simulink model "SAID"  (R2020a)
settings: Solver=ode45  StartTime=0  StopTime=15  FixedStep=0.002  RelTol=1e-3  AbsTol=1e-6
libraries: simulink x2, Solver_SF x1
settings Model: ExtModeTrigMode=oneshot  ExtModeArmWhenConnect=off  Creator=ywata  LastModifiedBy=wcbos
settings SolverCC: AutoScaleAbsTol=off  AlgebraicLoopSolver=LineSearch
settings DataIOCC: SaveFormat=Array  ReturnWorkspaceOutputs=off  SignalLoggingName=sigsOut
settings OptimizationCC: BlockReduction=off  BooleanDataType=off  ExpressionDepthLimit=2147483647  LifeSpan=inf
settings DebuggingCC: SaveWithParameterizedLinksMsg=none  UnderspecifiedInitializationDetection=Classic  MergeDetectMultiDrivingBlocksExec=none  SignalResolutionControl=TryResolveAllWithWarning  MultiTaskDSMMsg=warning  MultiTaskCondExecSysMsg=none  FcnCallInpInsideContextMsg=warning  StateNameClashWarn=warning  SFUnexpectedBacktrackingDiag=warning  SFNoUnconditionalDefaultTransitionDiag=warning  SFExecutionAtInitializationDiag=none  ArithmeticOperatorsInVariantConditions=warning
settings HardwareCC: ProdBitPerPointer=32  ProdBitPerSizeT=32  ProdBitPerPtrDiffT=32  ProdLargestAtomicFloat=None  ProdIntDivRoundTo=Undefined  ProdEndianess=Unspecified  ProdWordSize=32  ProdHWDeviceType=32-bit Generic  TargetUnknown=on
settings ModelReferenceCC: PropagateSignalLabelsOutOfModel=off
settings SFSimCC: SimUseLocalCustomCode=off  CustomCodeUndefinedFunction=UseInterfaceOnly
settings RTWCC: TemplateMakefile=grt_vc.tmf  RTWUseLocalCustomCode=off
settings CodeAppCC: StateflowObjectComments=on
settings GRTTargetCC: TargetFcnLib=ansi_tfl_tmw.mat  TargetLangStandard=C89/C90 (ANSI)  CombineOutputUpdateFcns=off  GRTInterface=on
settings ConfigComp: CovMetricSettings=dw  CovHtmlReporting=on  CovSaveCumulativeToWorkspaceVar=on  CovSaveSingleToWorkspaceVar=on  CovExternalEMLEnable=off

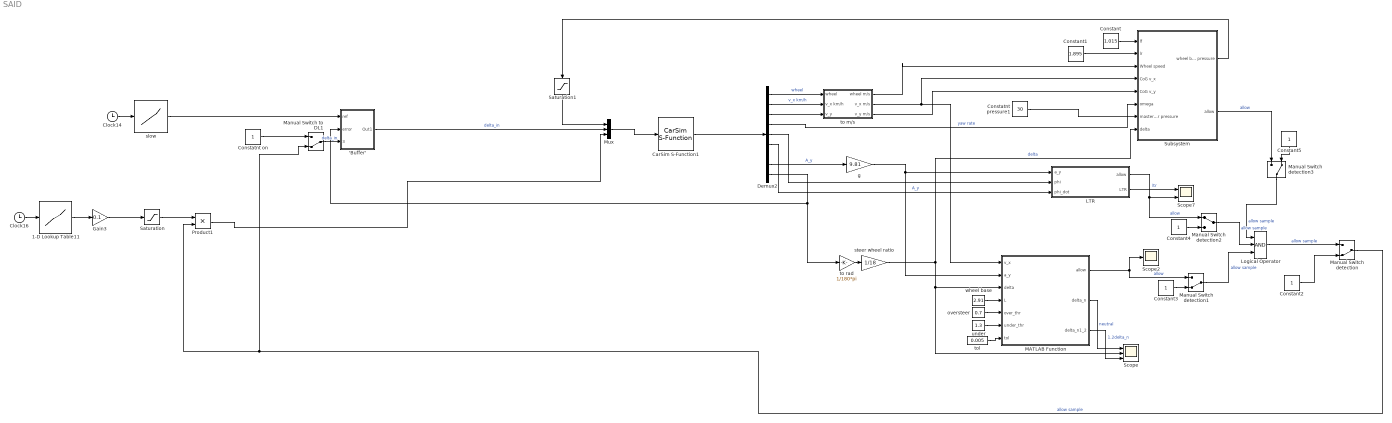
== system SAID ==
  'Buffer' : Subsystem
  1-D Lookup Table11 : Lookup_n-D  NumberOfTableDimensions=1  BreakpointsForDimension1=[0 2.9 linspace(3,25,length((cos(pi:0.01:2*pi)+1)/2))]  Table=[0 0 (cos(pi:0.01:2*pi)+1)/2]  ExtrapMethod=Clip  InternalRulePriority=Speed  RndMeth=Simplest  InputSameDT=on
  CarSim S-Function1 : Solver_SF/CarSim S-Function  Priority=1  SIMFILE=simfile.sim
  Clock14 : Clock
  Clock16 : Clock
  Constant : Constant  Value=1.015
  Constant1 : Constant  Value=1.895
  Constant{2..5} (4 alike) : Constant
  Constatnt on : Constant
  Constatnt pressure1 : Constant  Value=30
  Demux2 : Demux  Outputs=[4 1 1 1 1 1 1 1 1]
      settings: DisplayOption=none
  Gain3 : Gain  Gain=0.1
  LTR : Subsystem  mask{LTRthre=0.6, l_s=1.675, h=0.9345, h_m=0.9345, m=1870, k_s=130000, b_s=6000}
      mask prompts: LTRthre "LTR threshold"; l_s "Tack"; h "Height of roll centre to CoG"; h_m "Height of mass"; m "Mass"; k_s "suspension stiffness"; b_s "suspension damping coefficient"
  Logical Operator : Logic  Inputs=3  AllPortsSameDT=off  OutDataTypeStr=boolean
  MATLAB Function : MATLAB Function  TreatAsAtomicUnit=on
  Manual Switch detection : ManualSwitch  CurrentSetting=0
  Manual Switch detection1 : ManualSwitch  CurrentSetting=0
  Manual Switch detection2 : ManualSwitch
  Manual Switch detection3 : ManualSwitch  CurrentSetting=0
  Manual Switch to DL1 : ManualSwitch  CurrentSetting=0
  Mux : Mux  Inputs=[4 1 1]
  Product1 : Product
  Saturation : Saturate  UpperLimit=1  LowerLimit=0
  Saturation1 : Saturate  UpperLimit=30  LowerLimit=0
  Scope : Scope  NumInputPorts=3
  Scope2 : Scope
  Scope7 : Scope  NumInputPorts=2
  Subsystem : Subsystem
  g : Gain  Gain=9.81
  oversteer : Constant  Value=0.7
  slow : Lookup_n-D  NumberOfTableDimensions=1  BreakpointsForDimension1=[0 0.9 linspace(1,3,length((cos(pi:0.01:2*pi)+1)/2))]  Table=[0 0 (cos(pi:0.01:2*pi)+1)/2]  ExtrapMethod=Clip  InternalRulePriority=Speed  RndMeth=Simplest  InputSameDT=on
  steer wheel ratio : Gain  Gain=1/18
  to m/s : Subsystem
  to rad : Gain  Gain=1/180*pi
  tol : Constant  Value=0.005
  under : Constant  Value=1.3
  wheel base : Constant  Value=2.91
  wires:
  Demux2/2 -> to m/s/2(v_x km/h)  "v_x km/h"
  Mux/1 -> CarSim S-Function1/1
  'Buffer'/1(Out1) -> Mux/2  "delta_in"
  to rad/1 -> steer wheel ratio/1
  wheel base/1 -> MATLAB Function/4(L)
  g/1 -> LTR/1(a_y), MATLAB Function/2(a_y)
  oversteer/1 -> MATLAB Function/5(over_thr)
  under/1 -> MATLAB Function/6(under_thr)
  Demux2/8 -> g/1  "A_y"
  MATLAB Function/2(delta_n) -> Scope/1  "neutral"
  MATLAB Function/1(allow) -> Scope2/1, Manual Switch detection1/1  "allow"
  Demux2/9 -> to rad/1, 'Buffer'/2(error)
  tol/1 -> MATLAB Function/7(tol)
  Demux2/1 -> to m/s/1(wheel)  "wheel"
  Demux2/3 -> to m/s/3(v_y)
  to m/s/1(wheel m/s) -> Subsystem/3(Wheel speed)
  to m/s/2(v_x m/s) -> MATLAB Function/1(v_x), Subsystem/4(CoG v_x)
  to m/s/3(v_y m/s) -> Subsystem/5(CoG v_y)
  Demux2/4 -> Subsystem/6(omega)  "yaw rate"
  Constant/1 -> Subsystem/1(lf)
  Constant1/1 -> Subsystem/2(lr)
  Manual Switch detection/1 -> Product1/2, Manual Switch to DL1/2  "allow sample"
  Constant2/1 -> Manual Switch detection/2
  Constant3/1 -> Manual Switch detection1/2
  Manual Switch detection1/1 -> Logical Operator/3  "allow sample"
  Gain3/1 -> Saturation/1
  steer wheel ratio/1 -> MATLAB Function/3(delta), Scope/2, Subsystem/8(delta)  "delta"
  Saturation/1 -> Product1/1
  Constant4/1 -> Manual Switch detection2/2
  LTR/1(allow) -> Scope7/2, Manual Switch detection2/1  "allow"
  Manual Switch detection2/1 -> Logical Operator/2  "allow sample"
  Subsystem/2(allow) -> Manual Switch detection3/1  "allow"
  Constant5/1 -> Manual Switch detection3/2
  Manual Switch detection3/1 -> Logical Operator/1  "allow sample"
  LTR/2(LTR) -> Scope7/1  "ltr"
  Product1/1 -> Mux/3
  Logical Operator/1 -> Manual Switch detection/1  "allow sample"
  MATLAB Function/3(delta_n1_2) -> Scope/3  "1.2delta_n"
  Subsystem/1(wheel brake pressure) -> Saturation1/1
  Constatnt pressure1/1 -> Subsystem/7(master cylinder pressure)
  Clock16/1 -> 1-D Lookup Table11/1
  Demux2/5 -> LTR/2(phi)
  Demux2/6 -> LTR/3(phi_dot)  "A_y"
  Manual Switch to DL1/1 -> 'Buffer'/3(allow sample)  "delta_in"
  Constatnt on/1 -> Manual Switch to DL1/1
  CarSim S-Function1/1 -> Demux2/1
  Saturation1/1 -> Mux/1
  slow/1 -> 'Buffer'/1(ref)
  Clock14/1 -> slow/1
  1-D Lookup Table11/1 -> Gain3/1

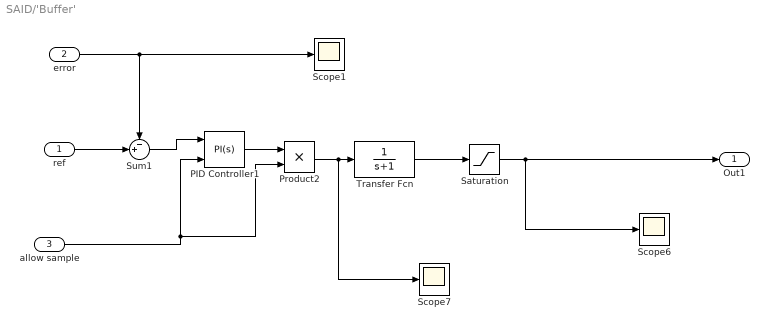
== system SAID/'Buffer' ==
  ref : Inport
  error : Inport  Port=2
  allow sample : Inport  Port=3
  PID Controller1 : simulink/Continuous/PID Controller  Controller=PI  Form=Parallel  TimeDomain=Continuous-time  UseExternalTs=off  SampleTime=-1  IntegratorMethod=Forward Euler  FilterMethod=Forward Euler  ControllerParametersSource=internal  P=17.6767934042104  I=4  D=0  UseFilter=on  N=745.731550681766  TunerSelectOption=Transfer Function Based (PID Tuner App)  InitialConditionSource=internal  InitialConditionForIntegrator=0  InitialConditionForFilter=0  DifferentiatorICPrevScaledInput=0  ExternalReset=either  TrackingMode=off  Kt=1  LimitOutput=on  UpperSaturationLimit=inf  LowerSaturationLimit=-inf  LinearizeAsGain=on  AntiWindupMode=clamping  Kb=1  POutMin=[]  POutMax=[]  IOutMin=[]  IOutMax=[]  DOutMin=[]  DOutMax=[]  NOutMin=[]  NOutMax=[]  SumOutMin=[]  SumOutMax=[]  SaturationOutMin=[]  SaturationOutMax=[]  PParamMin=[]  PParamMax=[]  IParamMin=[]  IParamMax=[]  DParamMin=[]  DParamMax=[]  NParamMin=[]  NParamMax=[]  KbParamMin=[]  KbParamMax=[]  KtParamMin=[]  KtParamMax=[]  KbOutMin=[]  KbOutMax=[]  KtOutMin=[]  KtOutMax=[]  IntegratorOutMin=[]  IntegratorOutMax=[]  FilterOutMin=[]  FilterOutMax=[]  SumI1OutMin=[]  SumI1OutMax=[]  SumI2OutMin=[]  SumI2OutMax=[]  SumI3OutMin=[]  SumI3OutMax=[]  SumI4OutMin=[]  SumI4OutMax=[]  SumDOutMin=[]  SumDOutMax=[]  DifferentiatorOutMin=[]  DifferentiatorOutMax=[]  FilterDiffOutCoefMin=[]  FilterDiffOutCoefMax=[]  ReciprocalOutMin=[]  ReciprocalOutMax=[]  SumDenOutMin=[]  SumDenOutMax=[]  SumNumOutMin=[]  SumNumOutMax=[]  DivideOutMin=[]  DivideOutMax=[]  UdiffTsProdOutMin=[]  UdiffTsProdOutMax=[]  NTsProdOutMin=[]  NTsProdOutMax=[]  UintegralTsProdOutMin=[]  UintegralTsProdOutMax=[]  UngainTsProdOutMin=[]  UngainTsProdOutMax=[]  IntegratorContinuousStateAttributes=''  IntegratorStateMustResolveToSignalObject=off  IntegratorRTWStateStorageClass=Auto  FilterContinuousStateAttributes=''  FilterStateMustResolveToSignalObject=off  FilterRTWStateStorageClass=Auto  ParallelPVariant=InternalParameters  IdealPVariant=Disabled  IVariant=InternalParameters  DVariant=Disabled  IntegratorVariant=Continuous  SatVariant=Enabled  AWVariant=ContClampingParallel  PCopyVariant=Disabled  TRVariant=Disabled  FdbkBlocksVariant=Forward  IdealPFdbkVariant=Disabled  SatFdbkVariant=Disabled  DerivativeFilterVariant=Disabled  NVariant=Disabled  NCopyVariant=Disabled_SignalSpec  FilterICVariant=Disabled  IntegratorICVariant=InternalICs  ExternalResetVariant=ExternalReset  TRSumVariant=Passthrough  SumFdbkVariant=Disabled  SumVariant=Sum_PI  TsampFilterVariant=InternalTs  TsampNgainVariant=Passthrough  TsampIntegralVariant=Passthrough
  Product2 : Product
  Saturation : Saturate  UpperLimit=360  LowerLimit=-360
  Scope1 : Scope
  Scope6 : Scope
  Scope7 : Scope
  Sum1 : Sum  Inputs=-+|
  Transfer Fcn : TransferFcn  Denominator=[1 1]
  Out1 : Outport
  wires:
  allow sample/1 -> Product2/2, PID Controller1/2
  ref/1 -> Sum1/2
  PID Controller1/1 -> Product2/1
  Saturation/1 -> Out1/1, Scope6/1
  Sum1/1 -> PID Controller1/1
  Transfer Fcn/1 -> Saturation/1
  error/1 -> Sum1/1, Scope1/1
  Product2/1 -> Scope7/1, Transfer Fcn/1

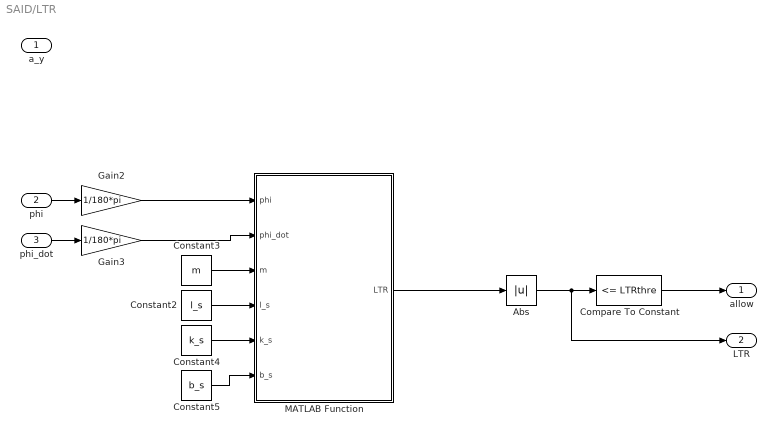
== system SAID/LTR ==
  a_y : Inport
  phi : Inport  Port=2
  phi_dot : Inport  Port=3
  Abs : Abs
  Compare To Constant : simulink/Logic and Bit Operations/Compare To Constant  relop=<=  const=LTRthre  OutDataTypeStr=boolean
  Constant2 : Constant  Value=l_s
  Constant3 : Constant  Value=m
  Constant4 : Constant  Value=k_s
  Constant5 : Constant  Value=b_s
  Gain2 : Gain  Gain=1/180*pi
  Gain3 : Gain  Gain=1/180*pi
  MATLAB Function : MATLAB Function  TreatAsAtomicUnit=on
  allow : Outport
  LTR : Outport  Port=2
  wires:
  Compare To Constant/1 -> allow/1
  Abs/1 -> LTR/1, Compare To Constant/1
  MATLAB Function/1(LTR) -> Abs/1
  Constant2/1 -> MATLAB Function/4(l_s)
  Constant3/1 -> MATLAB Function/3(m)
  phi/1 -> Gain2/1
  phi_dot/1 -> Gain3/1
  Gain2/1 -> MATLAB Function/1(phi)
  Gain3/1 -> MATLAB Function/2(phi_dot)
  Constant4/1 -> MATLAB Function/5(k_s)
  Constant5/1 -> MATLAB Function/6(b_s)

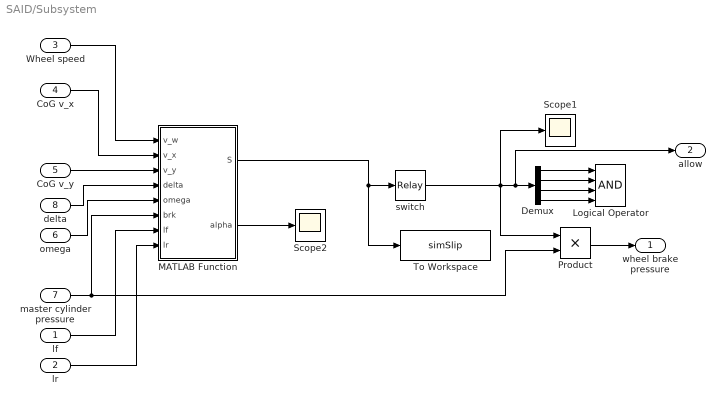
== system SAID/Subsystem ==
  lf : Inport
  lr : Inport  Port=2
  Wheel speed : Inport  Port=3
  CoG v_x : Inport  Port=4
  CoG v_y : Inport  Port=5
  omega : Inport  Port=6
  master cylinder pressure : Inport  Port=7
  delta : Inport  Port=8
  Demux : Demux
  Logical Operator : Logic  Inputs=4  AllPortsSameDT=off  OutDataTypeStr=boolean
  MATLAB Function : MATLAB Function  TreatAsAtomicUnit=on
  Product : Product
  Scope1 : Scope
  Scope2 : Scope
  To Workspace : ToWorkspace  VariableName=simSlip  SaveFormat=Timeseries  SampleTime=-1
  switch : Relay  OnSwitchValue=0.2  OffSwitchValue=0.1  OnOutputValue=0  OffOutputValue=1
  wheel brake pressure : Outport
  allow : Outport  Port=2
  wires:
  CoG v_x/1 -> MATLAB Function/2(v_x)
  Wheel speed/1 -> MATLAB Function/1(v_w)
  switch/1 -> Scope1/1, allow/1, Demux/1, Product/1
  master cylinder pressure/1 -> MATLAB Function/6(brk), Product/2
  Product/1 -> wheel brake pressure/1
  MATLAB Function/1(S) -> To Workspace/1, switch/1
  CoG v_y/1 -> MATLAB Function/3(v_y)
  delta/1 -> MATLAB Function/4(delta)
  omega/1 -> MATLAB Function/5(omega)
  lf/1 -> MATLAB Function/7(lf)
  lr/1 -> MATLAB Function/8(lr)
  Demux/1 -> Logical Operator/1
  Demux/2 -> Logical Operator/2
  Demux/3 -> Logical Operator/3
  Demux/4 -> Logical Operator/4
  MATLAB Function/2(alpha) -> Scope2/1

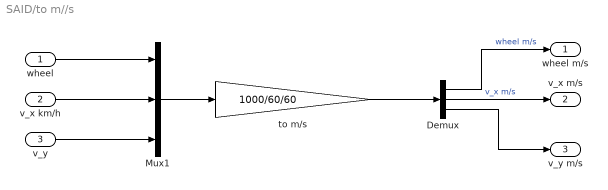
== system SAID/to m//s ==
  wheel : Inport
  v_x km/h : Inport  Port=2
  v_y : Inport  Port=3
  Demux : Demux  Outputs=[4 1 1]
  Mux1 : Mux  Inputs=[4 1 1]
  to m/s : Gain  Gain=1000/60/60
  wheel m/s : Outport
  v_x m/s : Outport  Port=2
  v_y m/s : Outport  Port=3
  wires:
  to m/s/1 -> Demux/1
  Demux/3 -> v_y m/s/1
  v_x km/h/1 -> Mux1/2
  Mux1/1 -> to m/s/1
  Demux/2 -> v_x m/s/1  "v_x m/s"
  wheel/1 -> Mux1/1
  Demux/1 -> wheel m/s/1  "wheel m/s"
  v_y/1 -> Mux1/3

== matlab function SAID/Subsystem/MATLAB Function ==
  data: v_w input; S output; v_x input; v_y input; delta input; omega input; brk input; lf input; lr input; alpha output
function [S, alpha] = tyreSlip(v_w, v_x, v_y, delta, omega, brk, lf, lr)
% brk = brake master cylinder pressure
% v in m/s
% omega in deg/s
% delta radian
%%
omega = deg2rad(omega);

theta = zeros(4,1);
alpha = zeros(4,1);

%%
% %% equation in book
% theta(1) =  atan((v_y + lf*omega)/v_x);
% theta(2) =  atan((v_y - lr*omega)/v_x);
% theta(3) =  theta(1);
% theta(4) =  theta(2);
% 
% alpha(1) = delta - theta(1);
% alpha(2) = - theta(2);
% alpha(3) = delta - theta(1);
% alpha(4) = - theta(4);
% 
% s_lat = tan(alpha);
% 
% if brk > 0.001 % braking
%     s_lon = (v_w - v_x)./v_x;
%     
% else
%     s_lon = (v_w - v_x)./v_w;
% end
% 
% S = sqrt(s_lat.^2 + s_lon.^2);

%% equation in paper

v = sqrt(v_x^2 + v_y^2);

theta(1) =  acos(max(min((v_x)/v, 0.999),-0.999));
theta(2) =  acos(max(min((v_x)/v, 0.999),-0.999));

% theta(1) =  asin((+ lf*omega)/v);
% theta(2) =  asin((- lr*omega)/v);

theta(3) =  theta(1);
theta(4) =  theta(2);

alpha(1) = delta - theta(1);
alpha(2) = - theta(2);
alpha(3) = delta - theta(1);
alpha(4) = - theta(4);

if brk > 0.001 % braking
    S = sqrt(v^2 + v_w.^2 - 2.*v.*v_w.*cos(alpha))/v;
    
else
    S = sqrt(v^2 + v_w.^2 - 2.*v.*v_w.*cos(alpha))./v_w;
end

if v_x < 1
    S = zeros(4,1);
end

== matlab function SAID/MATLAB Function ==
  data: v_x input; a_y input; delta input; L input; allow output; over_thr input; under_thr input; delta_n output; tol input; delta_n1_2 output
function [allow, delta_n, delta_n1_2] = ...
    neutralSteer(v_x, a_y, delta, L, over_thr, under_thr, tol)
% a_y m/s^2
% v_x m/s
% delta radian
% allow = 0 do not allow control signal to pass
% allow = 1 allow control signal to pass


if v_x < 0.01
    
    allow = 1;
    delta_n = 10000;
    if  delta > 0 && delta < delta_n*over_thr
        allow = 0;
    end
end

delta_n = L.*a_y./(v_x.^2);

delta_n1_2 = 1.2*delta_n;

if delta > 0
    %         delta_n = max(tol, delta_n);
    if (delta_n*over_thr > delta) || (delta > delta_n*under_thr)
        allow = 0;
    else
        allow = 1;
    end
else % delta is negative
    %         delta_n = min(-tol, delta_n);
    if (delta > delta_n*over_thr) || (delta < delta_n*under_thr)
        allow = 0;
    else
        allow = 1;
    end
end


if abs(abs(delta) - abs(2*delta_n)) < tol
    allow = 1;
end

== matlab function SAID/LTR/MATLAB Function ==
  data: phi input; LTR output; phi_dot input; m input; l_s input; k_s input; b_s input
function LTR = LTR_1dof_sim(phi, phi_dot, m, l_s, k_s, b_s)
g = 9.81;

LTR = (k_s*l_s .* sin(phi) + b_s*l_s .* phi_dot ...
    .* cos(phi)) / (m * g);

end
